simulink model "sim_SMC_algorithm_SMCtest"  (R2024b)
settings: Solver=FixedStepAuto  StartTime=0.0  StopTime=10.0  FixedStep=Tsim  RelTol=1e-3
InitFcn:
  | Tsim = 1e-4;
settings Model: Creator=Thu  LastModifiedBy=Lenovo
settings RTWCC: GPUComputeCapability=3.5

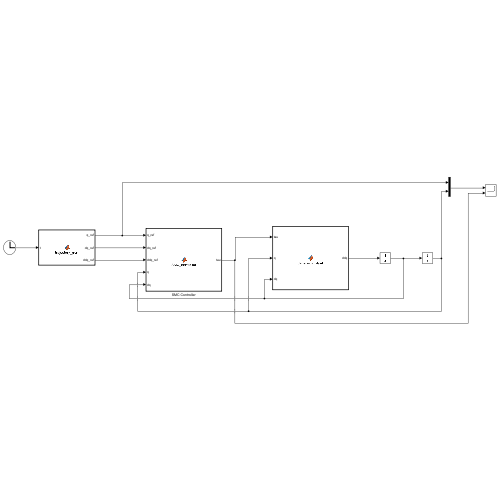
[thumbnail: Simulink's stored preview of the top-level diagram]
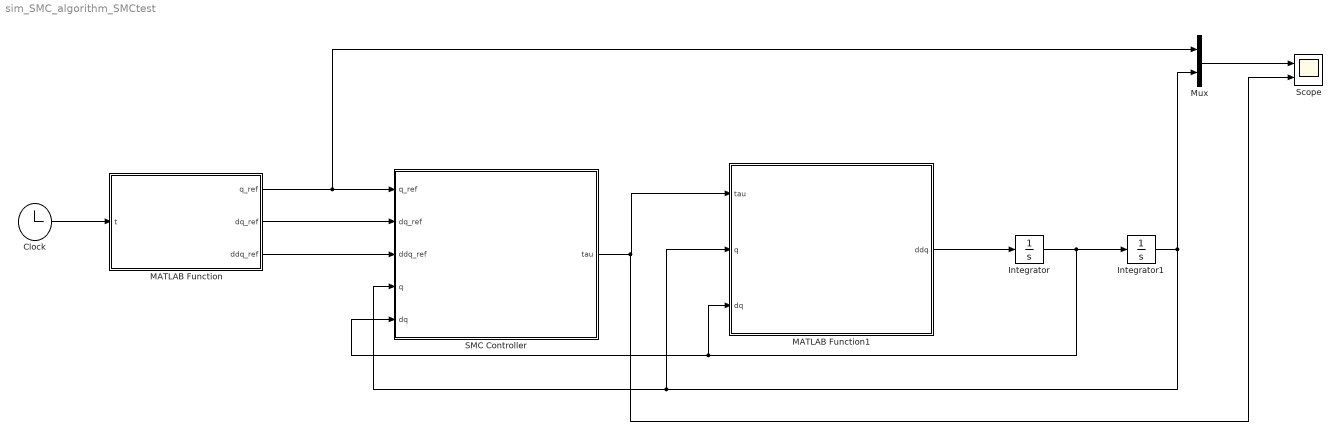
== system sim_SMC_algorithm_SMCtest ==
  Clock : Clock
  Integrator : Integrator  InitialCondition=[0; 0]
  Integrator1 : Integrator  InitialCondition=[0; 0]
  MATLAB Function : MATLAB Function  TreatAsAtomicUnit=on
  MATLAB Function1 : MATLAB Function  TreatAsAtomicUnit=on
  Mux : Mux  Inputs=2
  SMC Controller : MATLAB Function  TreatAsAtomicUnit=on
  Scope : Scope  NumInputPorts=2
  wires:
  MATLAB Function1/1(ddq) -> Integrator/1
  Integrator/1 -> SMC Controller/5(dq), MATLAB Function1/3(dq), Integrator1/1
  Integrator1/1 -> MATLAB Function1/2(q), SMC Controller/4(q), Mux/2
  MATLAB Function/1(q_ref) -> Mux/1, SMC Controller/1(q_ref)
  MATLAB Function/2(dq_ref) -> SMC Controller/2(dq_ref)
  MATLAB Function/3(ddq_ref) -> SMC Controller/3(ddq_ref)
  Clock/1 -> MATLAB Function/1(t)
  SMC Controller/1(tau) -> Scope/2, MATLAB Function1/1(tau)
  Mux/1 -> Scope/1

== matlab function sim_SMC_algorithm_SMCtest/MATLAB Function1 ==
  data: tau input; ddq output; q input; dq input
function ddq = dynamics_plant(tau, q, dq)
% 1. KHỞI TẠO KÍCH THƯỚC ĐẦU RA 
    ddq = zeros(2,1);

% ÉP KIỂU VECTOR CỘT
    tau = tau(:); q = q(:); dq = dq(:);
    
    q1 = q(1); q2 = q(2);
    dq1 = dq(1); dq2 = dq(2);

    % Ma trận Động lực học (Giữ nguyên như bên SMC)
    M = [cos(q2)/50 + 0.040128, cos(q2)/100 + 0.0066948;
         cos(q2)/100 + 0.0066948, 0.0066948];
         
    C = [dq2*sin(q2)*(-0.01),     sin(q2)*(dq1 + dq2)*(-0.01);
         (dq1*sin(q2))/100,       0];
         
    G = [cos(q1+q2)*0.4905 + cos(q1)*1.962;
         cos(q1+q2)*0.4905];

    % Giải phương trình động lực học tìm gia tốc thực tế
    % Dùng toán tử "\" (mldivide) của MATLAB thay cho inv(M) để hệ thống tính toán ổn định và nhanh hơn
    ddq = M \ (tau - C*dq - G); 
end

== matlab function sim_SMC_algorithm_SMCtest/SMC Controller ==
  data: q_ref input; tau output; dq_ref input; ddq_ref input; q input; dq input
function tau = SMC_controller(q_ref, dq_ref, ddq_ref, q, dq)
% 1. KHỞI TẠO KÍCH THƯỚC ĐẦU RA
    tau = zeros(2,1);    
    
% ÉP KIỂU VECTOR CỘT [2x1] (Cực kỳ quan trọng trong Simulink)
    q_ref = q_ref(:); dq_ref = dq_ref(:); ddq_ref = ddq_ref(:);
    q = q(:); dq = dq(:);

    %% 1. Các thông số bộ điều khiển 
    lambda = [1 0; 0 10]; % Ma trận hệ số mặt trượt
    K = [1 0; 0 1];        % Độ lợi điều khiển 
    Phi = [0.1 0; 0 0.1];  % Bề dày lớp biên để chống rung 

    q1 = q(1); q2 = q(2);
    dq1 = dq(1); dq2 = dq(2);

    %% 2. Tính toán Ma trận Động lực học 
    M = [cos(q2)/50 + 0.040128, cos(q2)/100 + 0.0066948;
         cos(q2)/100 + 0.0066948, 0.0066948];

    C = [dq2*sin(q2)*(-0.01),     sin(q2)*(dq1 + dq2)*(-0.01);
         (dq1*sin(q2))/100,       0];

    G = [cos(q1+q2)*0.4905 + cos(q1)*1.962;
         cos(q1+q2)*0.4905];

    %% 3. Thuật toán SMC
    e = q - q_ref;      % Sai số vị trí
    de = dq - dq_ref;   % Sai số vận tốc
    s = de + lambda * e;

    % Điều khiển tương đương 
    tau_eq = M * (ddq_ref - lambda * de) + C * dq + G;

    % Điều khiển chuyển mạch (Dùng hàm Saturation vector hóa)
    phi_diag = diag(Phi); % Trích xuất phần tử đường chéo [0.1; 0.1]
    sat_s = max(min(s ./ phi_diag, 1), -1); % Ràng buộc giá trị trong khoảng [-1, 1]

    tau_reach = -M * K * sat_s;

    %% 4. Đầu ra mô-men xoắn
    tau = tau_eq + tau_reach;
end

== matlab function sim_SMC_algorithm_SMCtest/MATLAB Function ==
  data: t input; q_ref output; dq_ref output; ddq_ref output
function [q_ref, dq_ref, ddq_ref] = trajectory_gen(t)
    % Tạo quỹ đạo thử nghiệm (Hàm Lượng giác)
    % Ví dụ: Khớp háng dao động 0.5 rad, khớp gối dao động 0.3 rad với tần số 1 Hz
    
    A1 = 0.5; w1 = 2 * pi * 1.0; 
    A2 = 0.3; w2 = 2 * pi * 1.0;
    
    % Vị trí mong muốn
    q_ref = [A1 * sin(w1 * t); 
             A2 * sin(w2 * t)];
             
    % Vận tốc mong muốn (Đạo hàm bậc 1)
    dq_ref = [A1 * w1 * cos(w1 * t); 
              A2 * w2 * cos(w2 * t)];
              
    % Gia tốc mong muốn (Đạo hàm bậc 2)
    ddq_ref = [-A1 * w1^2 * sin(w1 * t); 
               -A2 * w2^2 * sin(w2 * t)];
end
